simulink model "FOC_Chinh_luu_Bien_tan_IM_LC"  (R2017b)
settings: Solver=ode23tb  StartTime=0  StopTime=7  RelTol=1e-4  EnableMultiTasking=on
undefined symbols (not defined in the file or in its folder): DiscIntNeverNeededParam, sigbuilder_block
libraries: powerlib x38, simulink x4
settings Model: Creator=MinhTri  LastModifiedBy=chemi
settings DataIOCC: LimitDataPoints=on  SaveFormat=Array  SignalLoggingSaveFormat=ModelDataLogs
settings OptimizationCC: ExpressionDepthLimit=2147483647  LifeSpan=inf
settings DebuggingCC: UnderspecifiedInitializationDetection=Classic  MergeDetectMultiDrivingBlocksExec=none  SolverPrmCheckMsg=warning  FcnCallInpInsideContextMsg=warning  StateNameClashWarn=warning  SFUnexpectedBacktrackingDiag=warning  SFNoUnconditionalDefaultTransitionDiag=warning  SFExecutionAtInitializationDiag=none
settings HardwareCC: ProdBitPerPointer=32  ProdBitPerSizeT=32  ProdBitPerPtrDiffT=32  ProdLargestAtomicFloat=None  ProdIntDivRoundTo=Undefined  ProdEndianess=Unspecified  ProdWordSize=32  ProdHWDeviceType=32-bit Generic
settings ModelReferenceCC: PropagateSignalLabelsOutOfModel=off
settings SFSimCC: SimParseCustomCode=off
settings CodeAppCC: StateflowObjectComments=on
settings GRTTargetCC: TargetLangStandard=C89/C90 (ANSI)  GeneratePreprocessorConditionals=Disable all  CombineOutputUpdateFcns=off  GRTInterface=on
settings ConfigComp: CovMetricSettings=dw  CovHtmlReporting=on  CovSaveCumulativeToWorkspaceVar=on  CovSaveSingleToWorkspaceVar=on  CovExternalEMLEnable=off  CovSFcnEnable=off
settings SimscapeCC: SimscapeNormalizeSystem=off

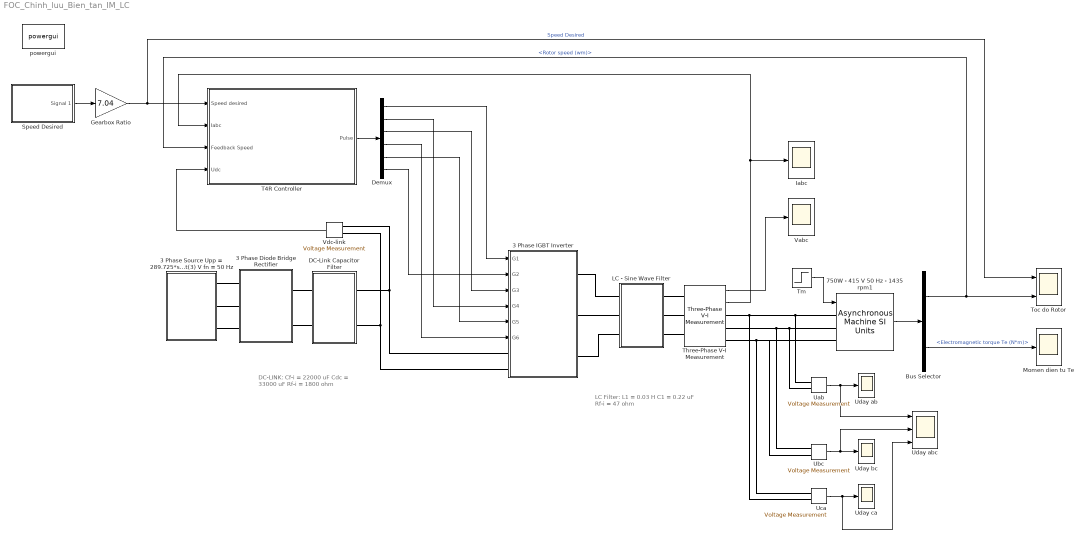
== system FOC_Chinh_luu_Bien_tan_IM_LC ==
  note: DC-LINK:
      |
      | Cf-i = 22000 uF
      | Cdc = 33000 uF
      | Rf-i = 1800 ohm
  note: LC Filter:
      | L1 = 0.03 H
      | C1 = 0.22 uF
      | Rf-i = 47 ohm
  3 Phase Diode Bridge Rectifier : Subsystem
  3 Phase IGBT Inverter : Subsystem
  3 Phase Source Upp = 289.725*sqrt(3) V fn = 50 Hz : Subsystem
  750W - 415 V 50 Hz - 1435 rpm1 : powerlib/Machines/Asynchronous Machine SI Units  RotorType=Squirrel-cage  PresetModel=No  MechanicalLoad=Torque Tm  ShowDetailedParameters=on  ReferenceFrame=Rotor  Units=SI  MeasurementBus=off  NominalParameters=[750 415 50]  Stator=[15.2 0.0255]  Rotor=[8.3 0.035]  Cage1=[ 0.022 0.226/377]  Cage2=[ 0.022 0.226/377]  Lm=0.57  Mechanical=[0.0214 0.0041 2]  PolePairs=2  InitialConditions="[ 1,0   0,0,0   0,0,0 ]"  SimulateSaturation=off  Saturation=[14.03593122, 27.81365428, 53.79336849, 72.68890987, 97.98006896, 148.6815601, 215.7428561, 302.9841135, 428.7778367 ; 230, 322, 414, 460, 506, 552, 598, 644, 690]  LoadFlowParameters=0  TsPowergui=0  TsBlock=-1  IterativeModel=Forward Euler  IterativeDiscreteModel=Trapezoidal non iterative  Pmec=0
  Bus Selector : BusSelector  OutputSignals=Mechanical.Rotor speed (wm),Mechanical.Electromagnetic torque Te (N*m)
  DC-Link Capacitor Filter : Subsystem
  Demux : Demux  Outputs=6
  Gearbox Ratio : Gain  Gain=7.04
  Iabc : Scope
  LC - Sine Wave Filter : Subsystem
  Momen dien tu Te : Scope
  Speed Desired : Subsystem  Tag=STV Subsys  LoadFcn=sigbuilder_block('load');  StartFcn=sigbuilder_block('start');  StopFcn=sigbuilder_block('stop');  ClipboardFcn=sigbuilder_block('clipboard');  mask(Sigbuilder block){tuvar=[0:10]}
      mask help: Simulink:masks:SigbuilderBlock_MD
      mask init:
      | if ~strcmp(get_param(bdroot(gcbh),'SimulationStatus'),'stopped') tuvar = sigbuilder_block('maskInit'); end
      settings: CopyFcn=sigbuilder_block('copy');  DeleteFcn=sigbuilder_block('delete');  ModelCloseFcn=sigbuilder_block('modelClose');  PreSaveFcn=sigbuilder_block('preSave');  PauseFcn=sigbuilder_block('pause');  ContinueFcn=sigbuilder_block('continue');  NameChangeFcn=sigbuilder_block('namechange');  OpenFcn=sigbuilder_block('open',[283.5 152.25 550.5 359.25 ]);  CloseFcn=sigbuilder_block('close');
      mask Display: plot(0, 0, 100, 100,[2, 2, 32, 32, 2], [68, 8, 8, 68, 68],[32, 2], [38, 38], [32, 19, 2],[53, 60, 44], [32, 17, 17, 2],[16, 16, 31, 31]);txt = getActiveGroup(gcbh);text(2, 100, txt,'verticalAlignment', 'top');
  T4R Controller : Subsystem
  Three-Phase V-I Measurement : powerlib/Measurements/Three-Phase V-I Measurement  VoltageMeasurement=phase-to-phase  SetLabelV=off  LabelV=Vabc  Vpu=off  VpuLL=off  CurrentMeasurement=yes  SetLabelI=off  LabelI=Iabc  Ipu=off  Pbase=100e6  Vbase=500e3  OutputType=Complex  PhasorSimulation=off  PSBequivalent=0
  Tm : Step  Time=0.5  After=5  SampleTime=0
  Toc do Rotor : Scope  NumInputPorts=2
  Uab : powerlib/Measurements/Voltage Measurement  PhasorSimulation=off  OutputType=Complex  PSBequivalent=0
  Ubc : powerlib/Measurements/Voltage Measurement  PhasorSimulation=off  OutputType=Complex  PSBequivalent=0
  Uca : powerlib/Measurements/Voltage Measurement  PhasorSimulation=off  OutputType=Complex  PSBequivalent=0
  Uday ab : Scope
  Uday abc : Scope  NumInputPorts=3
  Uday bc : Scope
  Uday ca : Scope
  Vabc : Scope
  Vdc-link : powerlib/Measurements/Voltage Measurement  PhasorSimulation=off  OutputType=Complex  PSBequivalent=0
  powergui : powerlib/powergui  Priority=1  SimulationMode=Continuous  SampleTime=0.001  frequency=60  Iterations=50  frequencyindice=50  Pbase=100e6  ErrMax=1e-4  UnitsV=kV  UnitsW=MW  buscounter=0  FunctionMessages=off  echomessages=off  EnableUseOfTLC=off  CurrentSourceSwitches=on  DisableSnubberDevices=off  DisableRonSwitches=off  DisableVfSwitches=off  DisplayEquations=off  SolverType=Backward Euler  Interpol=off  ExternalGateDelay=off  methode=off  Ts=0  x0status=blocks  SPID=off  SwTol=0  HookPort=off  RestoreLinks=warning  ResistiveCurrentMeasurement=off  Frange=[0:2:500]  Ylog=off  Xlog=on  ShowGrid=off  save=off  variable=ZData  structure=0  ZoomFFT=on  StartTime=0.0  cycles=1  DisplayStyle=1  fundamental=60  FreqAxis=off  MaxFrequency=1000  frequencyindicesteady=1  RmsSteady=1  display=off
  wires:
  Demux/2 -> 3 Phase IGBT Inverter/4(G4)
  T4R Controller/1(Pulse) -> Demux/1
  Speed Desired/1(Signal 1) -> Gearbox Ratio/1
  Three-Phase V-I Measurement/1 -> Vabc/1
  Vdc-link/1 -> T4R Controller/4(Udc)
  Bus Selector/1 -> Toc do Rotor/2, T4R Controller/3(Feedback Speed)  "<Rotor speed (wm)>"
  Gearbox Ratio/1 -> Toc do Rotor/1, T4R Controller/1(Speed desired)  "Speed Desired"
  Demux/6 -> 3 Phase IGBT Inverter/2(G2)
  Demux/1 -> 3 Phase IGBT Inverter/1(G1)
  Tm/1 -> 750W - 415 V 50 Hz - 1435 rpm1/1
  Ubc/1 -> Uday abc/2, Uday bc/1
  Uca/1 -> Uday abc/3, Uday ca/1
  Three-Phase V-I Measurement/2 -> Iabc/1, T4R Controller/2(Iabc)
  Uab/1 -> Uday abc/1, Uday ab/1
  Demux/5 -> 3 Phase IGBT Inverter/5(G5)
  Demux/4 -> 3 Phase IGBT Inverter/6(G6)
  Demux/3 -> 3 Phase IGBT Inverter/3(G3)
  750W - 415 V 50 Hz - 1435 rpm1/1 -> Bus Selector/1
  Bus Selector/2 -> Momen dien tu Te/1  "<Electromagnetic torque Te (N*m)>"
  connections:
  Uab/LConn1 -- Three-Phase V-I Measurement/RConn1 -- Uca/LConn2 -- 750W - 415 V 50 Hz - 1435 rpm1/LConn1
  DC-Link Capacitor Filter/RConn1 -- 3 Phase IGBT Inverter/LConn1 -- Vdc-link/LConn1
  Uab/LConn2 -- Three-Phase V-I Measurement/RConn2 -- Ubc/LConn1 -- 750W - 415 V 50 Hz - 1435 rpm1/LConn2
  Uca/LConn1 -- Three-Phase V-I Measurement/RConn3 -- 750W - 415 V 50 Hz - 1435 rpm1/LConn3 -- Ubc/LConn2
  DC-Link Capacitor Filter/RConn2 -- 3 Phase IGBT Inverter/LConn2 -- Vdc-link/LConn2
  DC-Link Capacitor Filter/LConn2 -- 3 Phase Diode Bridge Rectifier/RConn2
  3 Phase Source Upp = 289.725*sqrt(3) V fn = 50 Hz/RConn2 -- 3 Phase Diode Bridge Rectifier/LConn2
  DC-Link Capacitor Filter/LConn1 -- 3 Phase Diode Bridge Rectifier/RConn1
  3 Phase Source Upp = 289.725*sqrt(3) V fn = 50 Hz/RConn3 -- 3 Phase Diode Bridge Rectifier/LConn3
  3 Phase Source Upp = 289.725*sqrt(3) V fn = 50 Hz/RConn1 -- 3 Phase Diode Bridge Rectifier/LConn1
  LC - Sine Wave Filter/RConn1 -- Three-Phase V-I Measurement/LConn1
  LC - Sine Wave Filter/RConn2 -- Three-Phase V-I Measurement/LConn2
  LC - Sine Wave Filter/RConn3 -- Three-Phase V-I Measurement/LConn3
  LC - Sine Wave Filter/LConn2 -- 3 Phase IGBT Inverter/RConn2
  LC - Sine Wave Filter/LConn1 -- 3 Phase IGBT Inverter/RConn1
  3 Phase IGBT Inverter/RConn3 -- LC - Sine Wave Filter/LConn3

== system FOC_Chinh_luu_Bien_tan_IM_LC/3 Phase Diode Bridge Rectifier ==
  D{1..6} (6 alike) : powerlib/Power Electronics/Diode  Ron=0.001  Lon=0  Vf=0  IC=0  UseSnubber=off  Rs=500  Cs=250e-9  Measurements=off
  In1 : PMIOPort  Port=1  Side=Left
  In2 : PMIOPort  Port=2  Side=Left
  In3 : PMIOPort  Port=3  Side=Left
  Out1 : PMIOPort  Port=4  Side=Right
  Out2 : PMIOPort  Port=5  Side=Right
  connections:
  D1/LConn1 -- In1/RConn1 -- D4/RConn1
  D5/LConn1 -- D2/RConn1 -- In3/RConn1
  D4/LConn1 -- Out2/RConn1 -- D2/LConn1 -- D6/LConn1
  D5/RConn1 -- Out1/RConn1 -- D3/RConn1 -- D1/RConn1
  D3/LConn1 -- In2/RConn1 -- D6/RConn1

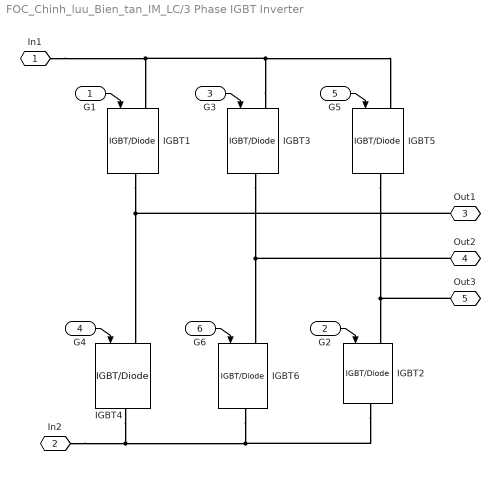
== system FOC_Chinh_luu_Bien_tan_IM_LC/3 Phase IGBT Inverter ==
  G1 : Inport
  G2 : Inport  Port=2
  G3 : Inport  Port=3
  G4 : Inport  Port=4
  G5 : Inport  Port=5
  G6 : Inport  Port=6
  IGBT{1..6} (6 alike) : powerlib/Power Electronics/IGBT//Diode  Ron=1e-3  Rs=1e5  Cs=inf  Measurements=off
  In1 : PMIOPort  Port=1  Side=Left
  In2 : PMIOPort  Port=2  Side=Left
  Out1 : PMIOPort  Port=3  Side=Right
  Out2 : PMIOPort  Port=4  Side=Right
  Out3 : PMIOPort  Port=5  Side=Right
  wires:
  G3/1 -> IGBT3/1
  G1/1 -> IGBT1/1
  G2/1 -> IGBT2/1
  G4/1 -> IGBT4/1
  G6/1 -> IGBT6/1
  G5/1 -> IGBT5/1
  connections:
  IGBT3/LConn1 -- IGBT5/LConn1 -- IGBT1/LConn1 -- In1/RConn1
  IGBT4/RConn1 -- In2/RConn1 -- IGBT6/RConn1 -- IGBT2/RConn1
  IGBT5/RConn1 -- Out3/RConn1 -- IGBT2/LConn1
  IGBT1/RConn1 -- Out1/RConn1 -- IGBT4/LConn1
  IGBT3/RConn1 -- Out2/RConn1 -- IGBT6/LConn1

== system FOC_Chinh_luu_Bien_tan_IM_LC/3 Phase Source Upp = 289.725*sqrt(3) V fn = 50 Hz ==
  Ground1 : powerlib/Elements/Ground  LConnTagsString=a
  Upp = 289.725*sqrt(3) V fn = 50 Hz : powerlib/Electrical Sources/Three-Phase Programmable Voltage Source  PositiveSequence=[289.725*sqrt(3) 0 50]  VariationEntity=None  VariationType=Table of time-amplitude pairs  VariationTypeAlt=Step  VariationStep=0.5  VariationRate=10  VariationMagnitude=0.3  VariationFrequency=2  VariationTiming=[1 2]  VariationPhaseA=off  Amplitudes=[1 0.8 1.2 1.0]  TimeValues=[0 0.1 0.15 0.2]  HarmonicGeneration=off  HarmonicA=[3 0.2 -25 0]  HarmonicB=[2 0.15 35 2]  Timing="[0.05  3]"  BusType=swing  Pref=0  Qref=0  Qmin=-inf  Qmax=inf
  Phase-A : PMIOPort  Port=1  Side=Right
  Phase-B : PMIOPort  Port=2  Side=Right
  Phase-C : PMIOPort  Port=3  Side=Right
  connections:
  Upp = 289.725*sqrt(3) V fn = 50 Hz/RConn2 -- Phase-B/RConn1
  Upp = 289.725*sqrt(3) V fn = 50 Hz/RConn3 -- Phase-C/RConn1
  Ground1/LConn1 -- Upp = 289.725*sqrt(3) V fn = 50 Hz/LConn1
  Upp = 289.725*sqrt(3) V fn = 50 Hz/RConn1 -- Phase-A/RConn1

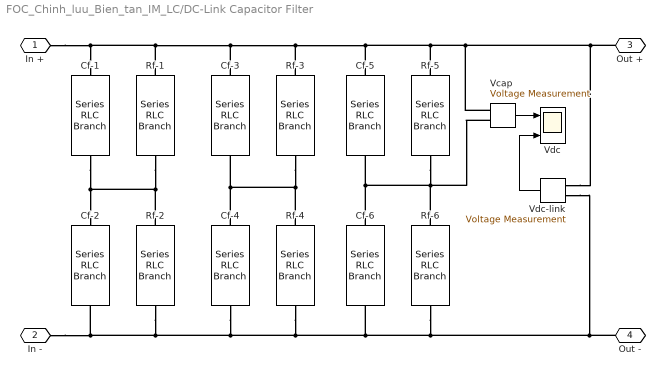
== system FOC_Chinh_luu_Bien_tan_IM_LC/DC-Link Capacitor Filter ==
  Cf-{1..6} (6 alike) : powerlib/Elements/Series RLC Branch  LConnTagsString=__new0  RConnTagsString=__new0  BranchType=C  Resistance=1  Inductance=1e-3  SetiL0=off  InitialCurrent=0  Capacitance=22000e-6  Setx0=off  InitialVoltage=0  Measurements=None
  Rf-{1..6} (6 alike) : powerlib/Elements/Series RLC Branch  LConnTagsString=__new0  RConnTagsString=__new0  BranchType=R  Resistance=1800  Inductance=1e-3  SetiL0=off  InitialCurrent=0  Capacitance=22000e-6  Setx0=off  InitialVoltage=0  Measurements=None
  Vcap : powerlib/Measurements/Voltage Measurement  PhasorSimulation=off  OutputType=Complex  PSBequivalent=0
  Vdc : Scope  NumInputPorts=2
  Vdc-link : powerlib/Measurements/Voltage Measurement  PhasorSimulation=off  OutputType=Complex  PSBequivalent=0
  In + : PMIOPort  Port=1  Side=Left
  In - : PMIOPort  Port=2  Side=Left
  Out + : PMIOPort  Port=3  Side=Right
  Out - : PMIOPort  Port=4  Side=Right
  wires:
  Vcap/1 -> Vdc/1
  Vdc-link/1 -> Vdc/2
  connections:
  Rf-3/RConn1 -- Cf-4/LConn1 -- Cf-3/RConn1 -- Rf-4/LConn1
  Cf-1/LConn1 -- Rf-1/LConn1 -- Cf-3/LConn1 -- Rf-3/LConn1 -- Out +/RConn1 -- Vdc-link/LConn1 -- Vcap/LConn1 -- Rf-5/LConn1 -- Cf-5/LConn1 -- In +/RConn1
  Rf-6/LConn1 -- Rf-5/RConn1 -- Vcap/LConn2 -- Cf-6/LConn1 -- Cf-5/RConn1
  Cf-1/RConn1 -- Cf-2/LConn1 -- Rf-2/LConn1 -- Rf-1/RConn1
  Rf-6/RConn1 -- Vdc-link/LConn2 -- Out -/RConn1 -- Cf-6/RConn1 -- Rf-4/RConn1 -- Cf-4/RConn1 -- Rf-2/RConn1 -- Cf-2/RConn1 -- In -/RConn1

== system FOC_Chinh_luu_Bien_tan_IM_LC/LC - Sine Wave Filter ==
  C1 : powerlib/Elements/Three-Phase Series RLC Branch  LConnTagsString=A|B|C  RConnTagsString=A|B|C  BranchType=C  Resistance=1  Inductance=0.03  Capacitance=0.22e-6  Measurements=None
  L1 : powerlib/Elements/Three-Phase Series RLC Branch  LConnTagsString=A|B|C  RConnTagsString=A|B|C  BranchType=L  Resistance=1  Inductance=0.03  Capacitance=1e-6  Measurements=None
  R1 : powerlib/Elements/Three-Phase Series RLC Branch  LConnTagsString=A|B|C  RConnTagsString=A|B|C  BranchType=R  Resistance=47  Inductance=0.03  Capacitance=0.22e-6  Measurements=None
  In1 : PMIOPort  Port=1  Side=Left
  In2 : PMIOPort  Port=2  Side=Left
  In3 : PMIOPort  Port=3  Side=Left
  Out1 : PMIOPort  Port=4  Side=Right
  Out2 : PMIOPort  Port=5  Side=Right
  Out3 : PMIOPort  Port=6  Side=Right
  connections:
  R1/RConn1 -- R1/RConn3 -- R1/RConn2
  L1/RConn1 -- C1/LConn1 -- Out1/RConn1
  R1/LConn1 -- C1/RConn1
  R1/LConn3 -- C1/RConn3
  R1/LConn2 -- C1/RConn2
  L1/RConn2 -- C1/LConn2 -- Out2/RConn1
  In3/RConn1 -- L1/LConn3
  In1/RConn1 -- L1/LConn1
  L1/LConn2 -- In2/RConn1
  L1/RConn3 -- Out3/RConn1 -- C1/LConn3

== system FOC_Chinh_luu_Bien_tan_IM_LC/Speed Desired ==
  Demux : Demux  Tag=STV Demux  Outputs=1
  FromWs : FromWorkspace  Tag=STV FromWs  VariableName=tuvar  SampleTime=0
      SigBuilderData=|
      | common.afterFinalStr = 'Extrapolate'
      | common.sampleTime = 0
      | dataSet.timeRange = [0 7]
      | dataSet.name = 'Group 1'
      | sbobj.Groups.Name = 'Group 1'
      | sbobj.Groups.Signals.Name = 'Signal 1'
      | sbobj.Groups.Signals.XData = [0 1 3 4 6 7]
      | sbobj.Groups.Signals.YData = [0 20 20 -20 -20 0]
      | sbobj.Groups.TimeRange = [0 7]
  Signal 1 : Outport  Tag=STV Outport
  wires:
  Demux/1 -> Signal 1/1
  FromWs/1 -> Demux/1

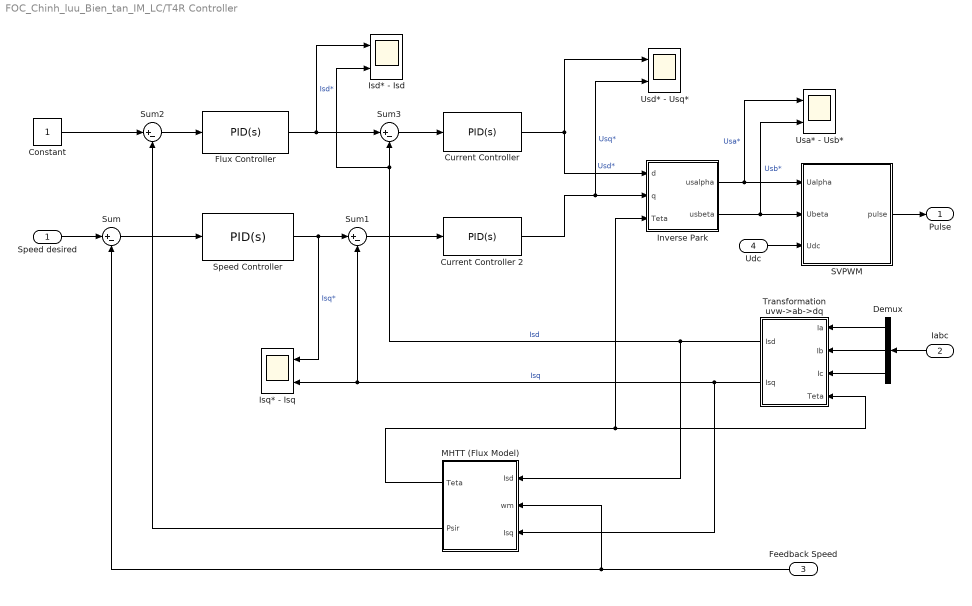
== system FOC_Chinh_luu_Bien_tan_IM_LC/T4R Controller ==
  Speed desired : Inport
  Iabc : Inport  Port=2
  Feedback Speed : Inport  Port=3
  Udc : Inport  Port=4
  Constant : Constant
  Current Controller : simulink/Continuous/PID Controller  Controller=PID  TimeDomain=Continuous-time  SampleTime=-1  IntegratorMethod=Forward Euler  FilterMethod=Forward Euler  Form=Parallel  UseFilter=on  ControllerParametersSource=internal  P=10  I=1  D=0  N=100  InitialConditionSource=internal  InitialConditionForIntegrator=0  InitialConditionForFilter=0  ExternalReset=none  LimitOutput=off  UpperSaturationLimit=inf  LowerSaturationLimit=-inf  LinearizeAsGain=on  AntiWindupMode=none  Kb=1  TrackingMode=off  Kt=1  PParamMin=[]  PParamMax=[]  IParamMin=[]  IParamMax=[]  DParamMin=[]  DParamMax=[]  NParamMin=[]  NParamMax=[]  KbParamMin=[]  KbParamMax=[]  KtParamMin=[]  KtParamMax=[]  POutMin=[]  POutMax=[]  IOutMin=[]  IOutMax=[]  DOutMin=[]  DOutMax=[]  NOutMin=[]  NOutMax=[]  KbOutMin=[]  KbOutMax=[]  KtOutMin=[]  KtOutMax=[]  IntegratorOutMin=[]  IntegratorOutMax=[]  FilterOutMin=[]  FilterOutMax=[]  SumOutMin=[]  SumOutMax=[]  SumI1OutMin=[]  SumI1OutMax=[]  SumI2OutMin=[]  SumI2OutMax=[]  SumI3OutMin=[]  SumI3OutMax=[]  SumDOutMin=[]  SumDOutMax=[]  SaturationOutMin=[]  SaturationOutMax=[]  IntegratorContinuousStateAttributes=''  IntegratorStateMustResolveToSignalObject=off  IntegratorRTWStateStorageClass=Auto  FilterContinuousStateAttributes=''  FilterStateMustResolveToSignalObject=off  FilterRTWStateStorageClass=Auto  DifferentiatorICPrevScaledInput=0  DifferentiatorOutMin=[]  DifferentiatorOutMax=[]  InitialConditionSetting=State (most efficient)  FilterDiffOutCoefMin=[]  FilterDiffOutCoefMax=[]  SumDenOutMin=[]  SumDenOutMax=[]  SumNumOutMin=[]  SumNumOutMax=[]  ReciprocalOutMin=[]  ReciprocalOutMax=[]  DivideOutMin=[]  DivideOutMax=[]  TunerSelectOption=Transfer Function Based (PID Tuner App)
  Current Controller 2 : simulink/Continuous/PID Controller  Controller=PID  TimeDomain=Continuous-time  SampleTime=-1  IntegratorMethod=Forward Euler  FilterMethod=Forward Euler  Form=Parallel  UseFilter=on  ControllerParametersSource=internal  P=10  I=1  D=0  N=100  InitialConditionSource=internal  InitialConditionForIntegrator=0  InitialConditionForFilter=0  ExternalReset=none  LimitOutput=off  UpperSaturationLimit=inf  LowerSaturationLimit=-inf  LinearizeAsGain=on  AntiWindupMode=none  Kb=1  TrackingMode=off  Kt=1  PParamMin=[]  PParamMax=[]  IParamMin=[]  IParamMax=[]  DParamMin=[]  DParamMax=[]  NParamMin=[]  NParamMax=[]  KbParamMin=[]  KbParamMax=[]  KtParamMin=[]  KtParamMax=[]  POutMin=[]  POutMax=[]  IOutMin=[]  IOutMax=[]  DOutMin=[]  DOutMax=[]  NOutMin=[]  NOutMax=[]  KbOutMin=[]  KbOutMax=[]  KtOutMin=[]  KtOutMax=[]  IntegratorOutMin=[]  IntegratorOutMax=[]  FilterOutMin=[]  FilterOutMax=[]  SumOutMin=[]  SumOutMax=[]  SumI1OutMin=[]  SumI1OutMax=[]  SumI2OutMin=[]  SumI2OutMax=[]  SumI3OutMin=[]  SumI3OutMax=[]  SumDOutMin=[]  SumDOutMax=[]  SaturationOutMin=[]  SaturationOutMax=[]  IntegratorContinuousStateAttributes=''  IntegratorStateMustResolveToSignalObject=off  IntegratorRTWStateStorageClass=Auto  FilterContinuousStateAttributes=''  FilterStateMustResolveToSignalObject=off  FilterRTWStateStorageClass=Auto  DifferentiatorICPrevScaledInput=0  DifferentiatorOutMin=[]  DifferentiatorOutMax=[]  InitialConditionSetting=State (most efficient)  FilterDiffOutCoefMin=[]  FilterDiffOutCoefMax=[]  SumDenOutMin=[]  SumDenOutMax=[]  SumNumOutMin=[]  SumNumOutMax=[]  ReciprocalOutMin=[]  ReciprocalOutMax=[]  DivideOutMin=[]  DivideOutMax=[]  TunerSelectOption=Transfer Function Based (PID Tuner App)
  Demux : Demux  Outputs=3
  "Flux Controller " : simulink/Continuous/PID Controller  Controller=PID  TimeDomain=Continuous-time  SampleTime=-1  IntegratorMethod=Forward Euler  FilterMethod=Forward Euler  Form=Parallel  UseFilter=on  ControllerParametersSource=internal  P=20  I=0.5  D=0  N=100  InitialConditionSource=internal  InitialConditionForIntegrator=0  InitialConditionForFilter=0  ExternalReset=none  LimitOutput=off  UpperSaturationLimit=inf  LowerSaturationLimit=-inf  LinearizeAsGain=on  AntiWindupMode=none  Kb=1  TrackingMode=off  Kt=1  PParamMin=[]  PParamMax=[]  IParamMin=[]  IParamMax=[]  DParamMin=[]  DParamMax=[]  NParamMin=[]  NParamMax=[]  KbParamMin=[]  KbParamMax=[]  KtParamMin=[]  KtParamMax=[]  POutMin=[]  POutMax=[]  IOutMin=[]  IOutMax=[]  DOutMin=[]  DOutMax=[]  NOutMin=[]  NOutMax=[]  KbOutMin=[]  KbOutMax=[]  KtOutMin=[]  KtOutMax=[]  IntegratorOutMin=[]  IntegratorOutMax=[]  FilterOutMin=[]  FilterOutMax=[]  SumOutMin=[]  SumOutMax=[]  SumI1OutMin=[]  SumI1OutMax=[]  SumI2OutMin=[]  SumI2OutMax=[]  SumI3OutMin=[]  SumI3OutMax=[]  SumDOutMin=[]  SumDOutMax=[]  SaturationOutMin=[]  SaturationOutMax=[]  IntegratorContinuousStateAttributes=''  IntegratorStateMustResolveToSignalObject=off  IntegratorRTWStateStorageClass=Auto  FilterContinuousStateAttributes=''  FilterStateMustResolveToSignalObject=off  FilterRTWStateStorageClass=Auto  DifferentiatorICPrevScaledInput=0  DifferentiatorOutMin=[]  DifferentiatorOutMax=[]  InitialConditionSetting=State (most efficient)  FilterDiffOutCoefMin=[]  FilterDiffOutCoefMax=[]  SumDenOutMin=[]  SumDenOutMax=[]  SumNumOutMin=[]  SumNumOutMax=[]  ReciprocalOutMin=[]  ReciprocalOutMax=[]  DivideOutMin=[]  DivideOutMax=[]  TunerSelectOption=Transfer Function Based (PID Tuner App)
  Inverse Park : Subsystem
  Isd* - Isd : Scope  NumInputPorts=2
  Isq* - Isq : Scope  NumInputPorts=2
  MHTT (Flux Model) : Subsystem
  SVPWM : Subsystem
  Speed Controller : simulink/Continuous/PID Controller  Controller=PID  TimeDomain=Continuous-time  SampleTime=-1  IntegratorMethod=Forward Euler  FilterMethod=Forward Euler  Form=Parallel  UseFilter=on  ControllerParametersSource=internal  P=20  I=0.5  D=0  N=0  InitialConditionSource=internal  InitialConditionForIntegrator=0  InitialConditionForFilter=0  ExternalReset=none  LimitOutput=off  UpperSaturationLimit=inf  LowerSaturationLimit=-inf  LinearizeAsGain=on  AntiWindupMode=none  Kb=1  TrackingMode=off  Kt=1  PParamMin=[]  PParamMax=[]  IParamMin=[]  IParamMax=[]  DParamMin=[]  DParamMax=[]  NParamMin=[]  NParamMax=[]  KbParamMin=[]  KbParamMax=[]  KtParamMin=[]  KtParamMax=[]  POutMin=[]  POutMax=[]  IOutMin=[]  IOutMax=[]  DOutMin=[]  DOutMax=[]  NOutMin=[]  NOutMax=[]  KbOutMin=[]  KbOutMax=[]  KtOutMin=[]  KtOutMax=[]  IntegratorOutMin=[]  IntegratorOutMax=[]  FilterOutMin=[]  FilterOutMax=[]  SumOutMin=[]  SumOutMax=[]  SumI1OutMin=[]  SumI1OutMax=[]  SumI2OutMin=[]  SumI2OutMax=[]  SumI3OutMin=[]  SumI3OutMax=[]  SumDOutMin=[]  SumDOutMax=[]  SaturationOutMin=[]  SaturationOutMax=[]  IntegratorContinuousStateAttributes=''  IntegratorStateMustResolveToSignalObject=off  IntegratorRTWStateStorageClass=Auto  FilterContinuousStateAttributes=''  FilterStateMustResolveToSignalObject=off  FilterRTWStateStorageClass=Auto  DifferentiatorICPrevScaledInput=0  DifferentiatorOutMin=[]  DifferentiatorOutMax=[]  InitialConditionSetting=State (most efficient)  FilterDiffOutCoefMin=[]  FilterDiffOutCoefMax=[]  SumDenOutMin=[]  SumDenOutMax=[]  SumNumOutMin=[]  SumNumOutMax=[]  ReciprocalOutMin=[]  ReciprocalOutMax=[]  DivideOutMin=[]  DivideOutMax=[]  TunerSelectOption=Transfer Function Based (PID Tuner App)
  Sum{,1..3} (4 alike) : Sum  Inputs=|+-
  Transformation uvw->ab->dq : Subsystem
  Usa* - Usb* : Scope  NumInputPorts=2
  Usd* - Usq* : Scope  NumInputPorts=2
  Pulse : Outport
  wires:
  Speed desired/1 -> Sum/1
  Sum/1 -> Speed Controller/1
  Constant/1 -> Sum2/1
  Sum2/1 -> "Flux Controller "/1
  Sum3/1 -> Current Controller/1
  Current Controller/1 -> Inverse Park/1(d), Usd* - Usq*/1  "Usd*"
  Inverse Park/1(usalpha) -> Usa* - Usb*/1, SVPWM/1(Ualpha)  "Usa*"
  Inverse Park/2(usbeta) -> Usa* - Usb*/2, SVPWM/2(Ubeta)  "Usb*"
  SVPWM/1(pulse) -> Pulse/1
  Feedback Speed/1 -> Sum/2, MHTT (Flux Model)/2(wm)
  Demux/1 -> Transformation uvw->ab->dq/1(Ia)
  Demux/2 -> Transformation uvw->ab->dq/2(Ib)
  Iabc/1 -> Demux/1
  Demux/3 -> Transformation uvw->ab->dq/3(Ic)
  MHTT (Flux Model)/1(Teta) -> Transformation uvw->ab->dq/4(Teta), Inverse Park/3(Teta)
  Transformation uvw->ab->dq/2(Isq) -> MHTT (Flux Model)/3(Isq), Sum1/2, Isq* - Isq/2  "Isq"
  Transformation uvw->ab->dq/1(Isd) -> Isd* - Isd/2, Sum3/2, MHTT (Flux Model)/1(Isd)  "Isd"
  Udc/1 -> SVPWM/3(Udc)
  Sum1/1 -> Current Controller 2/1
  Current Controller 2/1 -> Usd* - Usq*/2, Inverse Park/2(q)  "Usq*"
  "Flux Controller "/1 -> Sum3/1, Isd* - Isd/1  "Isd*"
  MHTT (Flux Model)/2(Psir) -> Sum2/2
  Speed Controller/1 -> Sum1/1, Isq* - Isq/1  "Isq*"

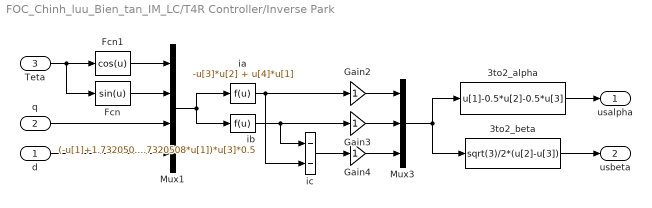
== system FOC_Chinh_luu_Bien_tan_IM_LC/T4R Controller/Inverse Park ==
  d : Inport
  q : Inport  Port=2
  Teta : Inport  Port=3
  3to2_alpha : Fcn  Expr=u[1]-0.5*u[2]-0.5*u[3]
  3to2_beta : Fcn  Expr=sqrt(3)/2*(u[2]-u[3])
  Fcn : Fcn  Expr=sin(u)
  Fcn1 : Fcn  Expr=cos(u)
  Gain2 : Gain  SaturateOnIntegerOverflow=on  OutDataTypeStr=Inherit: Same as input  ParamDataTypeStr=Inherit: Same as input
  Gain3 : Gain  SaturateOnIntegerOverflow=on  OutDataTypeStr=Inherit: Same as input  ParamDataTypeStr=Inherit: Same as input
  Gain4 : Gain  SaturateOnIntegerOverflow=on  OutDataTypeStr=Inherit: Same as input  ParamDataTypeStr=Inherit: Same as input
  Mux1 : Mux
  Mux3 : Mux  Inputs=3
  ia : Fcn  Expr=-u[3]*u[2] + u[4]*u[1]
  ib : Fcn  Expr=(-u[1]+1.7320508*u[2])*u[4]*0.5+(u[2]+1.7320508*u[1])*u[3]*0.5
  ic : Sum  Inputs=--  SaturateOnIntegerOverflow=on  InputSameDT=on  OutDataTypeStr=Inherit: Same as first input
  usalpha : Outport
  usbeta : Outport  Port=2
  wires:
  Fcn1/1 -> Mux1/1
  Teta/1 -> Fcn/1, Fcn1/1
  q/1 -> Mux1/3
  d/1 -> Mux1/4
  Gain3/1 -> Mux3/2
  ic/1 -> Gain4/1
  Gain4/1 -> Mux3/3
  Gain2/1 -> Mux3/1
  ia/1 -> Gain2/1, ic/2
  ib/1 -> Gain3/1, ic/1
  3to2_alpha/1 -> usalpha/1
  3to2_beta/1 -> usbeta/1
  Fcn/1 -> Mux1/2
  Mux1/1 -> ib/1, ia/1
  Mux3/1 -> 3to2_alpha/1, 3to2_beta/1

== system FOC_Chinh_luu_Bien_tan_IM_LC/T4R Controller/MHTT (Flux Model) ==
  Isd : Inport
  wm : Inport  Port=2
  Isq : Inport  Port=3
  Flux Observer : Subsystem  mask(Flux Calcultation){}
      mask init:
      | NF=0.44572610323020e-6;
      | DF=[1 -0.99998715486734];
  Teta Estimator : Subsystem
  Unit Delay : UnitDelay  SampleTime=0.0001
  Unit Delay1 : UnitDelay  SampleTime=0.0001
  Teta : Outport
  Psir : Outport  Port=2
  wires:
  Unit Delay1/1 -> Teta Estimator/3(Iq)
  Teta Estimator/1(Teta) -> Teta/1
  wm/1 -> Teta Estimator/2(wm)
  Isd/1 -> Unit Delay/1
  Unit Delay/1 -> Flux Observer/1(Id)
  Flux Observer/1(Phir) -> Teta Estimator/1(Phird), Psir/1
  Isq/1 -> Unit Delay1/1

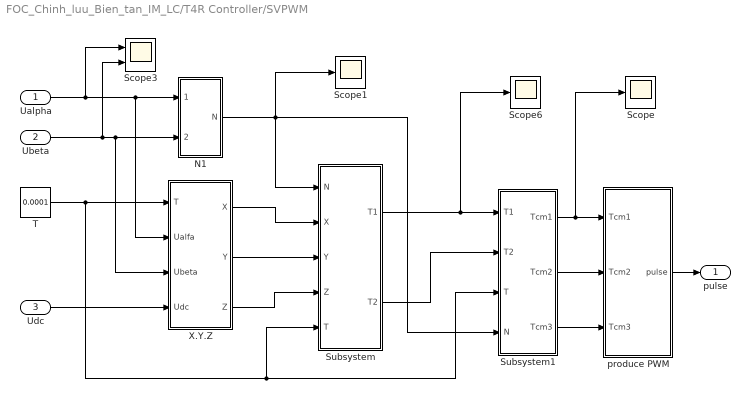
== system FOC_Chinh_luu_Bien_tan_IM_LC/T4R Controller/SVPWM ==
  Ualpha : Inport
  Ubeta : Inport  Port=2
  Udc : Inport  Port=3
  N1 : Subsystem
  Scope : Scope
  Scope1 : Scope
  Scope3 : Scope  NumInputPorts=2
  Scope6 : Scope
  Subsystem : Subsystem
  Subsystem1 : Subsystem
  T : Constant  Value=0.0001
  X.Y.Z : Subsystem
  produce PWM : Subsystem
  pulse : Outport
  wires:
  T/1 -> Subsystem1/3(T), Subsystem/5(T), X.Y.Z/1(T)
  Udc/1 -> X.Y.Z/4(Udc)
  N1/1(N) -> Subsystem/1(N), Subsystem1/4(N), Scope1/1
  X.Y.Z/1(X) -> Subsystem/2(X)
  X.Y.Z/2(Y) -> Subsystem/3(Y)
  X.Y.Z/3(Z) -> Subsystem/4(Z)
  Subsystem1/1(Tcm1) -> Scope/1, produce PWM/1(Tcm1)
  Subsystem1/2(Tcm2) -> produce PWM/2(Tcm2)
  Subsystem1/3(Tcm3) -> produce PWM/3(Tcm3)
  Ualpha/1 -> Scope3/1, X.Y.Z/2(Ualfa), N1/1(Ualpha)
  Subsystem/1(T1) -> Scope6/1, Subsystem1/1(T1)
  Subsystem/2(T2) -> Subsystem1/2(T2)
  Ubeta/1 -> X.Y.Z/3(Ubeta), N1/2(Ubeta), Scope3/2
  produce PWM/1(pulse) -> pulse/1

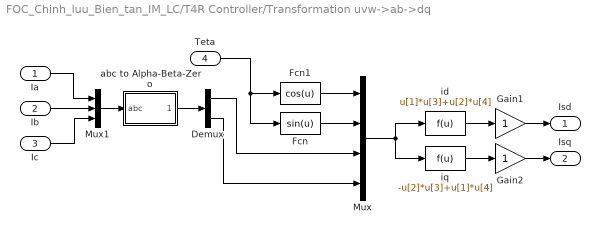
== system FOC_Chinh_luu_Bien_tan_IM_LC/T4R Controller/Transformation uvw->ab->dq ==
  Ia : Inport
  Ib : Inport  Port=2
  Ic : Inport  Port=3
  Teta : Inport  Port=4
  Demux : Demux  Outputs=2
  Fcn : Fcn  Expr=sin(u)
  Fcn1 : Fcn  Expr=cos(u)
  Gain1 : Gain  SaturateOnIntegerOverflow=on  OutDataTypeStr=Inherit: Same as input  ParamDataTypeStr=Inherit: Same as input
  Gain2 : Gain  SaturateOnIntegerOverflow=on  OutDataTypeStr=Inherit: Same as input  ParamDataTypeStr=Inherit: Same as input
  Mux : Mux
  Mux1 : Mux  Inputs=3
  abc to Alpha-Beta-Zero : Subsystem  AncestorBlock=powerlib_meascontrol/Transformations/abc to Alpha-Beta-Zero  DialogController=POWERSYS.PowerSysDialog  mask(abc to Alpha-Beta-Zero Transformation){}
      mask help: Perform a Clarke transformation from a three-phase (abc) signal to a alpha-beta-zero stationary reference frame.
      mask Help: helpview(psbhelp);
      mask Display:
      | plot([0 1], [0,1])
      | text(0.15,0.7,'abc')
      | text(0.55, 0.3,'\alpha\beta0','texmode','on')
  id : Fcn  Expr=u[1]*u[3]+u[2]*u[4]
  iq : Fcn  Expr=-u[2]*u[3]+u[1]*u[4]
  Isd : Outport
  Isq : Outport  Port=2
  wires:
  Ia/1 -> Mux1/1
  Ic/1 -> Mux1/3
  Mux1/1 -> abc to Alpha-Beta-Zero/1(abc)
  abc to Alpha-Beta-Zero/1(al_be) -> Demux/1
  Ib/1 -> Mux1/2
  Fcn/1 -> Mux/2
  Fcn1/1 -> Mux/1
  Mux/1 -> iq/1, id/1
  iq/1 -> Gain2/1
  id/1 -> Gain1/1
  Gain1/1 -> Isd/1
  Teta/1 -> Fcn/1, Fcn1/1
  Gain2/1 -> Isq/1
  Demux/1 -> Mux/3
  Demux/2 -> Mux/4

== system FOC_Chinh_luu_Bien_tan_IM_LC/T4R Controller/MHTT (Flux Model)/Flux Observer ==
  note: Phir = Lm *Id / (1 +Tr.s)
  note: Lm = 0.57 (H)
  note: Lr = Ll'r +Lm
      | = 0.035 + 0.57 = 0.605 (H)
  note: Tr = Lr / Rr
      | = 0.605/8.3 = 0.07289 (s)
  note: Rr = 8.3 ohms
  Id : Inport
  Discrete Tranfer Function : Subsystem  mask(First Order Low Pass Filter (Discrete)){T=0.07289, Ts=0.0001}
      mask prompts: T "Time constant T (s) :"; Ts "Time step (s)"
      mask help: H(s)=1/(1+T.s)
      mask init:
      | X=[0 1 2 3 4];
      |  Y=[-2 -2 -3 -4 -4];
      |  str=sprintf('\nH=1/(1+T.s)\n T= %g s\n\n\n',T);
      | num=1;
      | den=[T 1];
      | 
      | % discrete transfer function
      | % descending powers of z
      | numd= Ts/T;
      | dend=[ 1  (Ts-T)/T];
      mask Display:
      | plot(X,Y);
      | disp(str);
  Lm : Gain  Gain=0.57  SaturateOnIntegerOverflow=on  OutDataTypeStr=Inherit: Same as input  ParamDataTypeStr=Inherit: Same as input
  Phir : Outport
  wires:
  Discrete Tranfer Function/1(Out) -> Phir/1
  Id/1 -> Lm/1
  Lm/1 -> Discrete Tranfer Function/1(In)

== system FOC_Chinh_luu_Bien_tan_IM_LC/T4R Controller/MHTT (Flux Model)/Teta Estimator ==
  note: Teta= Electrical angle= integ ( wr + wm)
  note: wr = Rotor frequency (rad/s) = Lm *Iq / ( Tr * Phir)
  note: Lm = 0.57 (H)
  note: Rr= 8.3 ohms
  note: wm= Rotor mechanical speed (rad/s)
  note: Tr = Lr / Rr = 0.07289s
  note: Lr = Ll'r +Lm
      | = 0.035 + 0.57 = 0.605 (H)
  Phird : Inport
  wm : Inport  Port=2
  Iq : Inport  Port=3
  Discrete-Time Integrator : DiscreteIntegrator  SampleTime=0.0001  ICPrevOutput=DiscIntNeverNeededParam  ICPrevScaledInput=DiscIntNeverNeededParam
  Fcn : Fcn  Expr=0.57*u[1]/(u[2]*0.07289+1e-3)
  Gain2 : Gain  SaturateOnIntegerOverflow=on  OutDataTypeStr=Inherit: Same as input  ParamDataTypeStr=Inherit: Same as input
  Gain3 : Gain  Gain=2  SaturateOnIntegerOverflow=on  OutDataTypeStr=Inherit: Same as input  ParamDataTypeStr=Inherit: Same as input
  Mux1 : Mux  Inputs=2
  Sum : Sum  SaturateOnIntegerOverflow=on  InputSameDT=on  OutDataTypeStr=Inherit: Same as first input
  Teta : Outport  InitialOutput=0
  wires:
  Discrete-Time Integrator/1 -> Teta/1
  Sum/1 -> Discrete-Time Integrator/1
  Gain3/1 -> Sum/2
  Gain2/1 -> Sum/1
  wm/1 -> Gain3/1
  Fcn/1 -> Gain2/1
  Phird/1 -> Mux1/2
  Iq/1 -> Mux1/1
  Mux1/1 -> Fcn/1

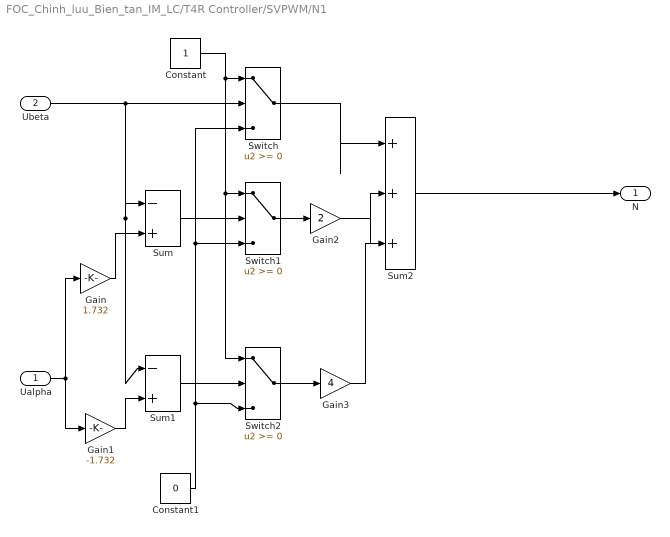
== system FOC_Chinh_luu_Bien_tan_IM_LC/T4R Controller/SVPWM/N1 ==
  Ualpha : Inport
  Ubeta : Inport  Port=2
  Constant : Constant
  Constant1 : Constant  Value=0
  Gain : Gain  Gain=1.732
  Gain1 : Gain  Gain=-1.732
  Gain2 : Gain  Gain=2
  Gain3 : Gain  Gain=4
  Sum : Sum  Inputs=|-+
  Sum1 : Sum  Inputs=|-+
  Sum2 : Sum  Inputs=|+++
  Switch : Switch
  Switch1 : Switch
  Switch2 : Switch
  N : Outport
  wires:
  Ubeta/1 -> Switch/2, Sum/1, Sum1/1
  Constant/1 -> Switch/1, Switch2/1, Switch1/1
  Ualpha/1 -> Gain1/1, Gain/1
  Gain/1 -> Sum/2
  Sum/1 -> Switch1/2
  Sum1/1 -> Switch2/2
  Gain1/1 -> Sum1/2
  Constant1/1 -> Switch/3, Switch1/3, Switch2/3
  Switch1/1 -> Gain2/1
  Switch2/1 -> Gain3/1
  Gain2/1 -> Sum2/2
  Switch/1 -> Sum2/1
  Gain3/1 -> Sum2/3
  Sum2/1 -> N/1

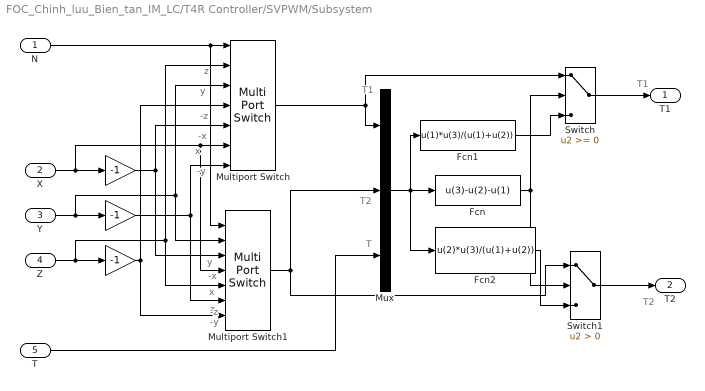
== system FOC_Chinh_luu_Bien_tan_IM_LC/T4R Controller/SVPWM/Subsystem ==
  note: z
  note: y
  note: -z
  note: -x
  note: x
  note: -y
  note: y
  note: -x
  note: x
  note: z
  note: -y
  note: -z
  note: T1
  note: T2
  note: T
  note: T1
  note: T2
  N : Inport
  X : Inport  Port=2
  Y : Inport  Port=3
  Z : Inport  Port=4
  T : Inport  Port=5
  " " : Gain  Gain=-1
  "  " : Gain  Gain=-1
  "    " : Gain  Gain=-1
  Fcn : Fcn  Expr=u(3)-u(2)-u(1)
  Fcn1 : Fcn  Expr=u(1)*u(3)/(u(1)+u(2))
  Fcn2 : Fcn  Expr=u(2)*u(3)/(u(1)+u(2))
  Multiport Switch : MultiPortSwitch  Inputs=6  DiagnosticForDefault=None
  Multiport Switch1 : MultiPortSwitch  Inputs=6  DiagnosticForDefault=None
  Mux : Mux  Inputs=3
  Switch : Switch
  Switch1 : Switch  Criteria=u2 > Threshold
  T1 : Outport
  T2 : Outport  Port=2
  wires:
  N/1 -> Multiport Switch1/1, Multiport Switch/1
  X/1 -> Multiport Switch1/4, Multiport Switch/6, " "/1
  Y/1 -> Multiport Switch1/2, Multiport Switch/3, "  "/1
  Z/1 -> Multiport Switch1/5, Multiport Switch/2, "    "/1
  "    "/1 -> Multiport Switch1/7, Multiport Switch/4
  "  "/1 -> Multiport Switch/7, Multiport Switch1/6
  " "/1 -> Multiport Switch/5, Multiport Switch1/3
  Multiport Switch/1 -> Mux/1, Switch/1
  Multiport Switch1/1 -> Switch1/1, Mux/2
  T/1 -> Mux/3
  Mux/1 -> Fcn/1, Fcn1/1, Fcn2/1
  Fcn/1 -> Switch/2, Switch1/2
  Fcn1/1 -> Switch/3
  Fcn2/1 -> Switch1/3
  Switch/1 -> T1/1
  Switch1/1 -> T2/1

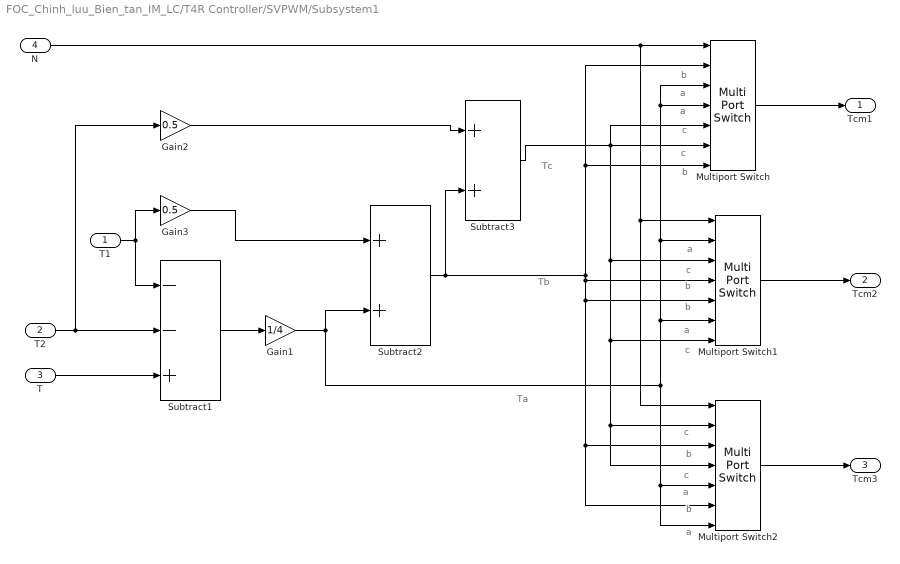
== system FOC_Chinh_luu_Bien_tan_IM_LC/T4R Controller/SVPWM/Subsystem1 ==
  note: Ta
  note: Tb
  note: Tc
  note: b
  note: a
  note: a
  note: c
  note: c
  note: b
  note: a
  note: c
  note: b
  note: b
  note: a
  note: c
  note: c
  note: b
  note: c
  note: a
  note: b
  note: a
  T1 : Inport
  T2 : Inport  Port=2
  T : Inport  Port=3
  N : Inport  Port=4
  Gain1 : Gain  Gain=1/4
  Gain2 : Gain  Gain=0.5
  Gain3 : Gain  Gain=0.5
  Multiport Switch : MultiPortSwitch  Inputs=6  DiagnosticForDefault=None
  Multiport Switch1 : MultiPortSwitch  Inputs=6  DiagnosticForDefault=None
  Multiport Switch2 : MultiPortSwitch  Inputs=6  DiagnosticForDefault=None
  Subtract1 : Sum  Inputs=--+
  Subtract2 : Sum
  Subtract3 : Sum
  Tcm1 : Outport
  Tcm2 : Outport  Port=2
  Tcm3 : Outport  Port=3
  wires:
  T2/1 -> Gain2/1, Subtract1/2
  T/1 -> Subtract1/3
  T1/1 -> Gain3/1, Subtract1/1
  Gain3/1 -> Subtract2/1
  Subtract1/1 -> Gain1/1
  Gain1/1 -> Subtract2/2, Multiport Switch/3, Multiport Switch/4, Multiport Switch1/2, Multiport Switch1/6, Multiport Switch2/5, Multiport Switch2/7
  Subtract2/1 -> Subtract3/2, Multiport Switch/2, Multiport Switch/7, Multiport Switch1/4, Multiport Switch1/5, Multiport Switch2/3, Multiport Switch2/6
  Gain2/1 -> Subtract3/1
  N/1 -> Multiport Switch/1, Multiport Switch2/1, Multiport Switch1/1
  Multiport Switch/1 -> Tcm1/1
  Multiport Switch1/1 -> Tcm2/1
  Multiport Switch2/1 -> Tcm3/1
  Subtract3/1 -> Multiport Switch/5, Multiport Switch/6, Multiport Switch1/3, Multiport Switch1/7, Multiport Switch2/2, Multiport Switch2/4

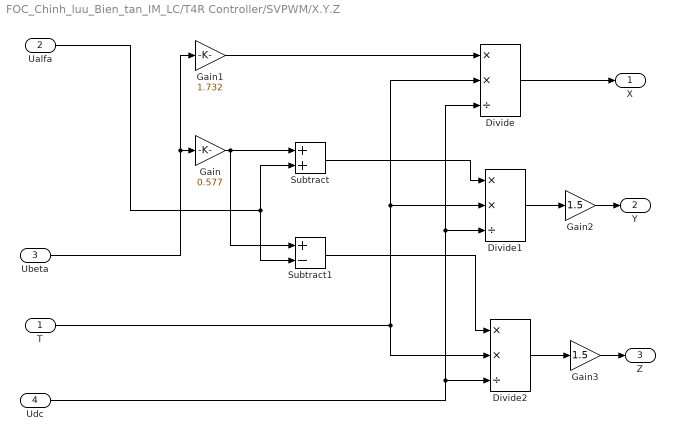
== system FOC_Chinh_luu_Bien_tan_IM_LC/T4R Controller/SVPWM/X.Y.Z ==
  T : Inport
  Ualfa : Inport  Port=2
  Ubeta : Inport  Port=3
  Udc : Inport  Port=4
  Divide : Product  Inputs=**/
  Divide1 : Product  Inputs=**/
  Divide2 : Product  Inputs=**/
  Gain : Gain  Gain=0.577
  Gain1 : Gain  Gain=1.732
  Gain2 : Gain  Gain=1.5
  Gain3 : Gain  Gain=1.5
  Subtract : Sum
  Subtract1 : Sum  Inputs=+-
  X : Outport
  Y : Outport  Port=2
  Z : Outport  Port=3
  wires:
  Gain/1 -> Subtract/1, Subtract1/1
  Gain1/1 -> Divide/1
  T/1 -> Divide2/2, Divide1/2, Divide/2
  Udc/1 -> Divide2/3, Divide1/3, Divide/3
  Ualfa/1 -> Subtract1/2, Subtract/2
  Subtract/1 -> Divide1/1
  Subtract1/1 -> Divide2/1
  Divide/1 -> X/1
  Divide1/1 -> Gain2/1
  Divide2/1 -> Gain3/1
  Gain2/1 -> Y/1
  Gain3/1 -> Z/1
  Ubeta/1 -> Gain1/1, Gain/1

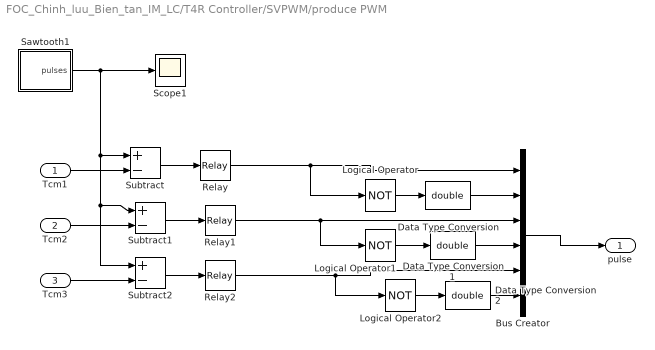
== system FOC_Chinh_luu_Bien_tan_IM_LC/T4R Controller/SVPWM/produce PWM ==
  Tcm1 : Inport
  Tcm2 : Inport  Port=2
  Tcm3 : Inport  Port=3
  Bus Creator : BusCreator  Inputs=6
  Data Type Conversion : DataTypeConversion  OutDataTypeStr=double
  Data Type Conversion1 : DataTypeConversion  OutDataTypeStr=double
  Data Type Conversion2 : DataTypeConversion  OutDataTypeStr=double
  Logical Operator : Logic  Operator=NOT  AllPortsSameDT=off
  Logical Operator1 : Logic  Operator=NOT  AllPortsSameDT=off
  Logical Operator2 : Logic  Operator=NOT  AllPortsSameDT=off
  Relay : Relay
  Relay1 : Relay
  Relay2 : Relay
  Sawtooth1 : Subsystem
  Scope1 : Scope
  Subtract : Sum  Inputs=+-
  Subtract1 : Sum  Inputs=+-
  Subtract2 : Sum  Inputs=+-
  pulse : Outport
  wires:
  Subtract/1 -> Relay/1
  Subtract1/1 -> Relay1/1
  Subtract2/1 -> Relay2/1
  Sawtooth1/1(pulses) -> Subtract/1, Subtract2/1, Subtract1/1, Scope1/1
  Tcm1/1 -> Subtract/2
  Tcm2/1 -> Subtract1/2
  Tcm3/1 -> Subtract2/2
  Logical Operator1/1 -> Data Type Conversion1/1
  Logical Operator2/1 -> Data Type Conversion2/1
  Logical Operator/1 -> Data Type Conversion/1
  Relay/1 -> Bus Creator/1, Logical Operator/1
  Relay1/1 -> Bus Creator/3, Logical Operator1/1
  Relay2/1 -> Bus Creator/5, Logical Operator2/1
  Bus Creator/1 -> pulse/1
  Data Type Conversion/1 -> Bus Creator/2
  Data Type Conversion1/1 -> Bus Creator/4
  Data Type Conversion2/1 -> Bus Creator/6

== system FOC_Chinh_luu_Bien_tan_IM_LC/T4R Controller/Transformation uvw->ab->dq/abc to Alpha-Beta-Zero ==
  abc : Inport  PortDimensions=3
  Gain3 : Gain  Gain="[ 1   -1/2   -1/2; 0   sqrt(3)/2   -sqrt(3)/2]"  Multiplication=Matrix(K*u) (u vector)  SaturateOnIntegerOverflow=on  OutDataTypeStr=Inherit: Same as input  ParamDataTypeStr=Inherit: Same as input
  al_be : Outport
  wires:
  abc/1 -> Gain3/1
  Gain3/1 -> al_be/1

== system FOC_Chinh_luu_Bien_tan_IM_LC/T4R Controller/MHTT (Flux Model)/Flux Observer/Discrete Tranfer Function ==
  In : Inport
  Discrete Transfer Fcn : DiscreteTransferFcn  Numerator=numd  Denominator=dend  SampleTime=Ts
  Out : Outport  InitialOutput=0
  wires:
  Discrete Transfer Fcn/1 -> Out/1
  In/1 -> Discrete Transfer Fcn/1

== system FOC_Chinh_luu_Bien_tan_IM_LC/T4R Controller/SVPWM/produce PWM/Sawtooth1 ==
  Integrator : Integrator
  Pulse Generator : DiscretePulseGenerator  PulseType=Time based  Period=0.0001  PulseWidth=50
  Sum1 : Sum  Inputs=-+|  SaturateOnIntegerOverflow=on  InputSameDT=on  OutDataTypeStr=Inherit: Same as first input
  modulation index2 : Gain  Gain=2  SaturateOnIntegerOverflow=on  OutDataTypeStr=Inherit: Same as input  ParamDataTypeStr=Inherit: Same as input
  pi/1 : Constant
  pulses : Outport
  wires:
  pi/1/1 -> Sum1/1
  modulation index2/1 -> Sum1/2
  Sum1/1 -> Integrator/1
  Integrator/1 -> pulses/1
  Pulse Generator/1 -> modulation index2/1
